simulink model "FIR_32tap"  (Simulink 9.0)
settings: Solver=FixedStepDiscrete  StartTime=0.0  StopTime=1024*sample_time  RelTol=1e-3
PreLoadFcn:
  | FIR_32tap_setup
InitFcn:
  | FIR_32tap_setup
values from neighbouring files (symbols this model uses):
  sample_time = 1/clock_freq    (= 1e-08)    [FIR_32tap_setup.m]
settings Model: Creator=Vitaly  LastModifiedBy=HONOR
settings DataIOCC: SaveFormat=Dataset
settings OptimizationCC: LifeSpan=auto
settings DebuggingCC: UnderspecifiedInitializationDetection=Simplified  MergeDetectMultiDrivingBlocksExec=error  SFUnexpectedBacktrackingDiag=error  SFNoUnconditionalDefaultTransitionDiag=error  SFExecutionAtInitializationDiag=warning
settings HardwareCC: ProdBitPerPointer=64  ProdBitPerSizeT=64  ProdBitPerPtrDiffT=64  ProdLargestAtomicFloat=Float  ProdIntDivRoundTo=Zero  ProdEndianess=LittleEndian  ProdWordSize=64  ProdHWDeviceType=Intel->x86-64 (Windows64)
settings ModelReferenceCC: PropagateSignalLabelsOutOfModel=on
settings CodeAppCC: StateflowObjectComments=off
settings GRTTargetCC: TargetLangStandard=C99 (ISO)
settings ConfigComp: CovMetricSettings=dwe  CovHtmlReporting=off  CovSaveCumulativeToWorkspaceVar=off  CovSaveSingleToWorkspaceVar=off  CovExternalEMLEnable=on

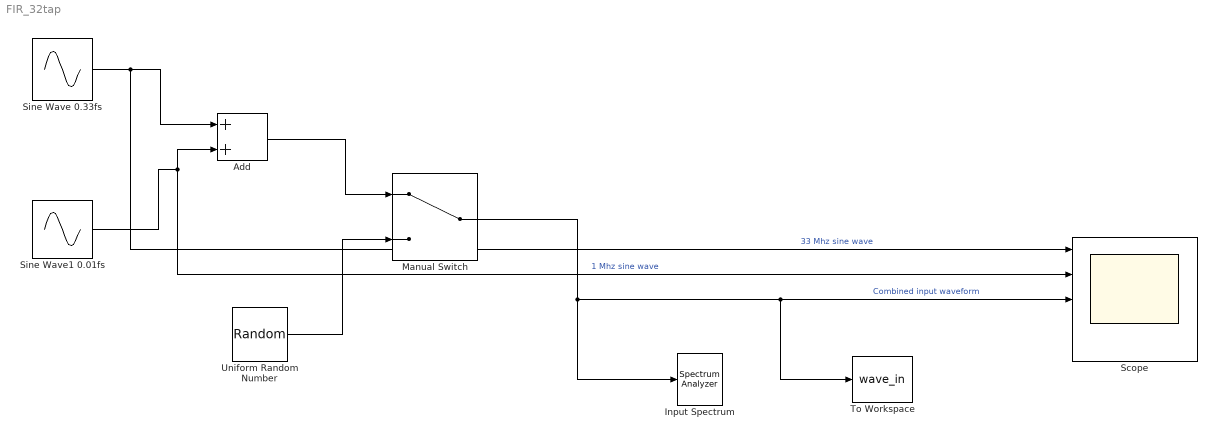
== system FIR_32tap ==
  Add : Sum
  Input Spectrum : SpectrumAnalyzer
  Manual Switch : ManualSwitch
  Scope : Scope  NumInputPorts=5
  "Sine Wave 0.33fs " : Sin  SineType=Sample based  Amplitude=2^9-1  Samples=3  SampleTime=sample_time
  Sine Wave1 0.01fs : Sin  SineType=Sample based  Amplitude=2^9-1  Samples=100  SampleTime=sample_time
  To Workspace : ToWorkspace  VariableName=wave_in  SampleTime=-1
      settings: MaxDataPoints=256
  Uniform Random Number : UniformRandomNumber  Minimum=-2^10  Maximum=2^10-1  SampleTime=sample_time
  wires:
  "Sine Wave 0.33fs "/1 -> Scope/1, Add/1  "33 Mhz sine wave"
  Sine Wave1 0.01fs/1 -> Scope/2, Add/2  "1 Mhz sine wave"
  Add/1 -> Manual Switch/1
  Uniform Random Number/1 -> Manual Switch/2
  Manual Switch/1 -> Input Spectrum/1, To Workspace/1, Scope/3  "Combined input waveform"
